simulink model "attitude_kalman_filter"  (R2023a)
settings: configuration reference "configuration_filter" (kept outside this file)
undefined symbols (not defined in the file): alignment_done_bool, dead_reckoning_bool, DiscIntNeverNeededParam, Eul_rad, filt, lin_acc_est_mDs2, rot_K_est_bias_OB_B_radDs, rot_K_est_OB_B_radDs, sfor_est_B_mDs, sfor_est_bias_B_mDs2, sim, x_est
libraries: lib_jacobians x5, lib_kinematics x4
settings Model: Creator=FC_dev1  LastModifiedBy=FC_dev1
settings ConfigSetRef: SourceName=configuration_filter  SourceLocation=Base Workspace

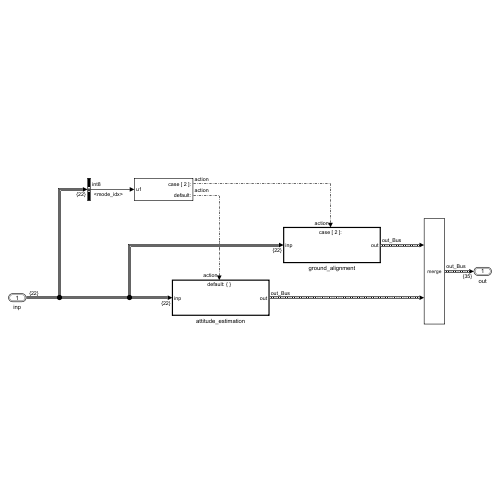
[thumbnail: Simulink's stored preview of the top-level diagram]
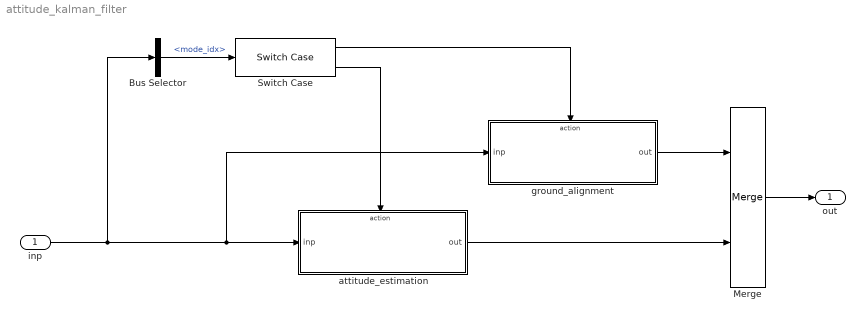
== system attitude_kalman_filter ==
  inp : Inport  OutDataTypeStr=Bus: inp_Bus
  Bus Selector : BusSelector  OutputSignals=mode_idx
  Merge : Merge
  Switch Case : SwitchCase  CaseConditions={filt.modes.ground_alignment}
  attitude_estimation : Subsystem
  ground_alignment : Subsystem
  out : Outport  OutDataTypeStr=Bus: out_Bus
  wires:
  inp/1 -> Bus Selector/1, attitude_estimation/1(inp), ground_alignment/1(inp)
  attitude_estimation/1(out) -> Merge/2
  Bus Selector/1 -> Switch Case/1  "<mode_idx>"
  Switch Case/1 -> ground_alignment/Action
  Switch Case/2 -> attitude_estimation/Action
  ground_alignment/1(out) -> Merge/1
  Merge/1 -> out/1

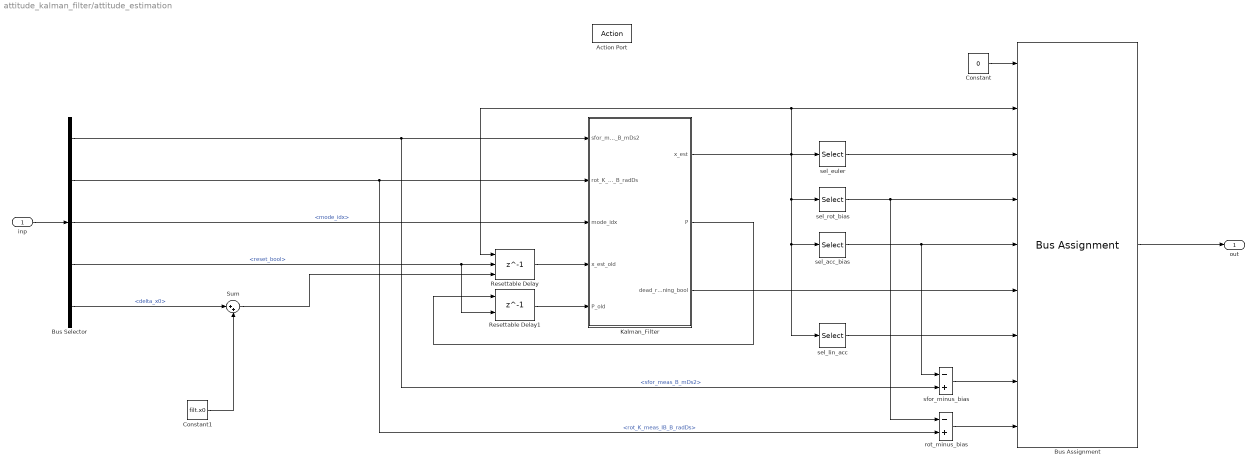
== system attitude_kalman_filter/attitude_estimation ==
  inp : Inport  OutDataTypeStr=Bus: inp_Bus
  Action Port : ActionPort  InitializeStates=reset  ActionPortLabel=default:
  Bus Assignment : BusAssignment  AssignedSignals=x_est,Eul_rad,rot_K_est_bias_OB_B_radDs,sfor_est_bias_B_mDs2,dead_reckoning_bool,lin_acc_est_mDs2,sfor_est_B_mDs,rot_K_est_OB_B_radDs
  Bus Selector : BusSelector  OutputSignals=sfor_meas_B_mDs2,rot_K_meas_IB_B_radDs,mode_idx,reset_bool,delta_x0
  Constant : Constant  Value=0  OutDataTypeStr=Bus: out_Bus
  Constant1 : Constant  Value=filt.x0  VectorParams1D=off
  Kalman_Filter : Subsystem
  Resettable Delay : Delay  DelayLength=1  InitialConditionSource=Input port  ExternalReset=Level hold
      settings: InputPortMap=u0,r5,p4
  Resettable Delay1 : Delay  DelayLength=1  InitialCondition=filt.P0  ExternalReset=Level hold
      settings: InputPortMap=u0,r5
  Sum : Sum  Inputs=|++
  rot_minus_bias : Sum  Inputs=-+
  sel_acc_bias : Selector  NumberOfDimensions=2  InputPortWidth=3  IndexOptions=Index vector (dialog),Index vector (dialog)  Indices=filt.acc_bias_idx,1  OutputSizes=1,1
  sel_euler : Selector  NumberOfDimensions=2  InputPortWidth=3  IndexOptions=Index vector (dialog),Index vector (dialog)  Indices=filt.eul_idx,1  OutputSizes=1,1
  sel_lin_acc : Selector  NumberOfDimensions=2  InputPortWidth=3  IndexOptions=Index vector (dialog),Index vector (dialog)  Indices=filt.lin_acc_idx,1  OutputSizes=1,1
  sel_rot_bias : Selector  NumberOfDimensions=2  InputPortWidth=3  IndexOptions=Index vector (dialog),Index vector (dialog)  Indices=filt.rot_bias_idx,1  OutputSizes=1,1
  sfor_minus_bias : Sum  Inputs=-+
  out : Outport  OutDataTypeStr=Bus: out_Bus
  wires:
  Bus Selector/1 -> sfor_minus_bias/2, Kalman_Filter/1(sfor_meas_B_mDs2)  "<sfor_meas_B_mDs2>"
  rot_minus_bias/1 -> Bus Assignment/9
  sel_acc_bias/1 -> sfor_minus_bias/1, Bus Assignment/5
  sel_rot_bias/1 -> rot_minus_bias/1, Bus Assignment/4
  Bus Selector/2 -> rot_minus_bias/2, Kalman_Filter/2(rot_K_meas_IB_B_radDs)  "<rot_K_meas_IB_B_radDs>"
  Constant/1 -> Bus Assignment/1
  Bus Selector/3 -> Kalman_Filter/3(mode_idx)  "<mode_idx>"
  sel_euler/1 -> Bus Assignment/3
  Kalman_Filter/1(x_est) -> sel_lin_acc/1, sel_acc_bias/1, sel_rot_bias/1, Resettable Delay/1, Bus Assignment/2, sel_euler/1
  Bus Assignment/1 -> out/1
  sel_lin_acc/1 -> Bus Assignment/7
  sfor_minus_bias/1 -> Bus Assignment/8
  Kalman_Filter/3(dead_reckoning_bool) -> Bus Assignment/6
  inp/1 -> Bus Selector/1
  Resettable Delay1/1 -> Kalman_Filter/5(P_old)
  Resettable Delay/1 -> Kalman_Filter/4(x_est_old)
  Bus Selector/4 -> Resettable Delay1/2, Resettable Delay/2  "<reset_bool>"
  Bus Selector/5 -> Sum/1  "<delta_x0>"
  Kalman_Filter/2(P) -> Resettable Delay1/1
  Sum/1 -> Resettable Delay/3
  Constant1/1 -> Sum/2

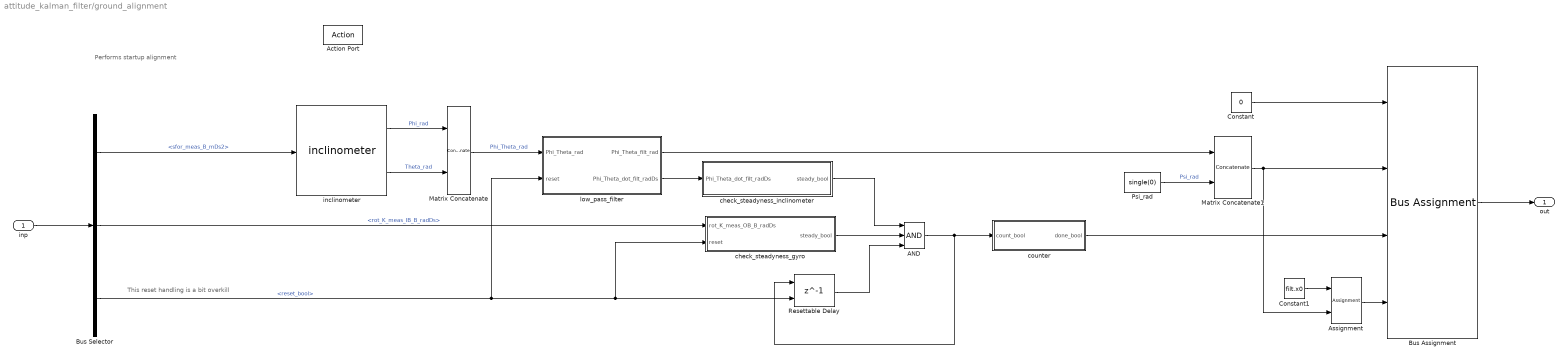
== system attitude_kalman_filter/ground_alignment ==
  note: Performs startup alignment
  note: This reset handling is a bit overkill
  inp : Inport  OutDataTypeStr=Bus: inp_Bus
  Action Port : ActionPort  InitializeStates=reset  ActionPortLabel=case [ 2 ]:
  AND : Logic  Inputs=3  AllPortsSameDT=off  OutDataTypeStr=boolean
  Assignment : Assignment  NumberOfDimensions=2  DiagnosticForDimensions=Warning  IndexOptions=Index vector (dialog),Index vector (dialog)  Indices=filt.eul_idx,1  OutputSizes=1,1
  Bus Assignment : BusAssignment  AssignedSignals=Eul_rad,alignment_done_bool,x_est
  Bus Selector : BusSelector  OutputSignals=sfor_meas_B_mDs2,rot_K_meas_IB_B_radDs,reset_bool
  Constant : Constant  Value=0  OutDataTypeStr=Bus: out_Bus
  Constant1 : Constant  Value=filt.x0  VectorParams1D=off
  Matrix Concatenate : Concatenate  Mode=Multidimensional array
  Matrix Concatenate1 : Concatenate  Mode=Multidimensional array
  Psi_rad : Constant  Value=single(0)
  Resettable Delay : Delay  DelayLength=1  InitialCondition=false  ExternalReset=Level
      settings: InputPortMap=u0,r5
  check_steadyness_gyro : Subsystem
  check_steadyness_inclinometer : Subsystem
  counter : Subsystem
  inclinometer : lib_kinematics/inclinometer  SystemSampleTime=-1  VariantActivationTime=update diagram  Latency=0  AutoFrameSizeCalculation=off
  low_pass_filter : Subsystem
  out : Outport  OutDataTypeStr=Bus: out_Bus
  wires:
  inp/1 -> Bus Selector/1
  Bus Assignment/1 -> out/1
  Constant/1 -> Bus Assignment/1
  Bus Selector/1 -> inclinometer/1  "<sfor_meas_B_mDs2>"
  inclinometer/2 -> Matrix Concatenate/2  "Theta_rad"
  inclinometer/1 -> Matrix Concatenate/1  "Phi_rad"
  Psi_rad/1 -> Matrix Concatenate1/2  "Psi_rad"
  Matrix Concatenate/1 -> low_pass_filter/1(Phi_Theta_rad)  "Phi_Theta_rad"
  low_pass_filter/1(Phi_Theta_filt_rad) -> Matrix Concatenate1/1
  Matrix Concatenate1/1 -> Bus Assignment/2, Assignment/2
  low_pass_filter/2(Phi_Theta_dot_filt_radDs) -> check_steadyness_inclinometer/1(Phi_Theta_dot_filt_radDs)
  Bus Selector/2 -> check_steadyness_gyro/1(rot_K_meas_OB_B_radDs)  "<rot_K_meas_IB_B_radDs>"
  check_steadyness_inclinometer/1(steady_bool) -> AND/1
  check_steadyness_gyro/1(steady_bool) -> AND/2
  AND/1 -> counter/1(count_bool), Resettable Delay/1
  counter/1(done_bool) -> Bus Assignment/3
  Bus Selector/3 -> low_pass_filter/2(reset), check_steadyness_gyro/2(reset), Resettable Delay/2  "<reset_bool>"
  Resettable Delay/1 -> AND/3
  Assignment/1 -> Bus Assignment/4
  Constant1/1 -> Assignment/1

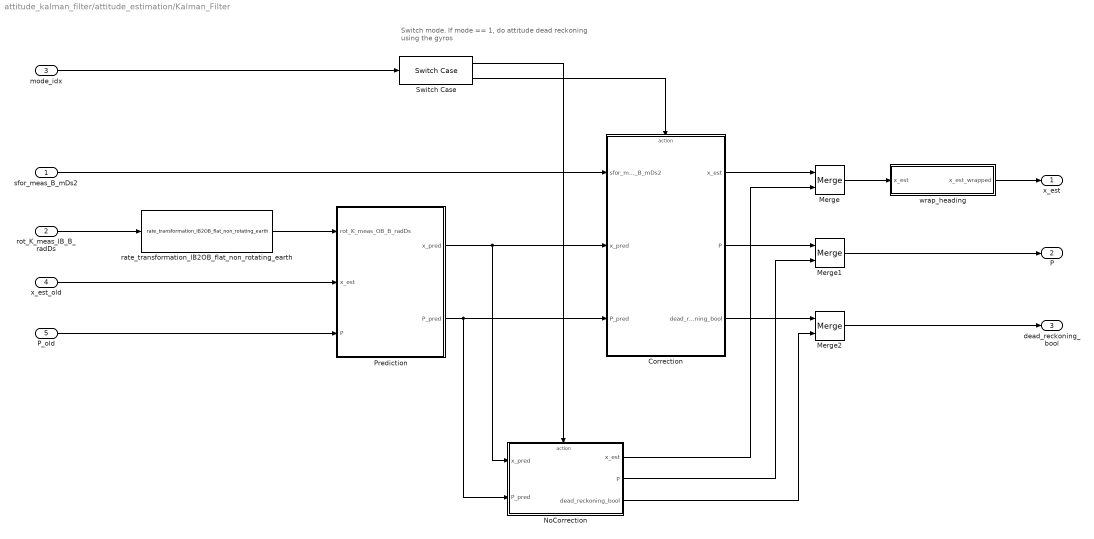
== system attitude_kalman_filter/attitude_estimation/Kalman_Filter ==
  note: Switch mode.
      | If mode == 1, do attitude dead reckoning using the gyros
  sfor_meas_B_mDs2 : Inport
  rot_K_meas_IB_B_radDs : Inport  Port=2
  mode_idx : Inport  Port=3
  x_est_old : Inport  Port=4
  P_old : Inport  Port=5
  Correction : Subsystem
  Merge : Merge
  Merge1 : Merge
  Merge2 : Merge
  NoCorrection : Subsystem
  Prediction : Subsystem
  Switch Case : SwitchCase  CaseConditions={filt.modes.dead_reckoning}
  rate_transformation_IB2OB_flat_non_rotating_earth : lib_kinematics/rate_transformation_IB2OB_flat_non_rotating_earth  SystemSampleTime=-1  VariantActivationTime=update diagram  Latency=0  AutoFrameSizeCalculation=off
  wrap_heading : Subsystem
  x_est : Outport
  P : Outport  Port=2
  dead_reckoning_bool : Outport  Port=3
  wires:
  Prediction/2(P_pred) -> Correction/3(P_pred), NoCorrection/2(P_pred)
  x_est_old/1 -> Prediction/2(x_est)
  Correction/2(P) -> Merge1/1
  sfor_meas_B_mDs2/1 -> Correction/1(sfor_meas_B_mDs2)
  Prediction/1(x_pred) -> NoCorrection/1(x_pred), Correction/2(x_pred)
  rot_K_meas_IB_B_radDs/1 -> rate_transformation_IB2OB_flat_non_rotating_earth/1
  Correction/1(x_est) -> Merge/1
  P_old/1 -> Prediction/3(P)
  mode_idx/1 -> Switch Case/1
  Switch Case/1 -> NoCorrection/Action
  Merge/1 -> wrap_heading/1(x_est)
  Merge1/1 -> P/1
  Switch Case/2 -> Correction/Action
  NoCorrection/1(x_est) -> Merge/2
  NoCorrection/2(P) -> Merge1/2
  Merge2/1 -> dead_reckoning_bool/1
  Correction/3(dead_reckoning_bool) -> Merge2/1
  NoCorrection/3(dead_reckoning_bool) -> Merge2/2
  rate_transformation_IB2OB_flat_non_rotating_earth/1 -> Prediction/1(rot_K_meas_OB_B_radDs)
  wrap_heading/1(x_est_wrapped) -> x_est/1

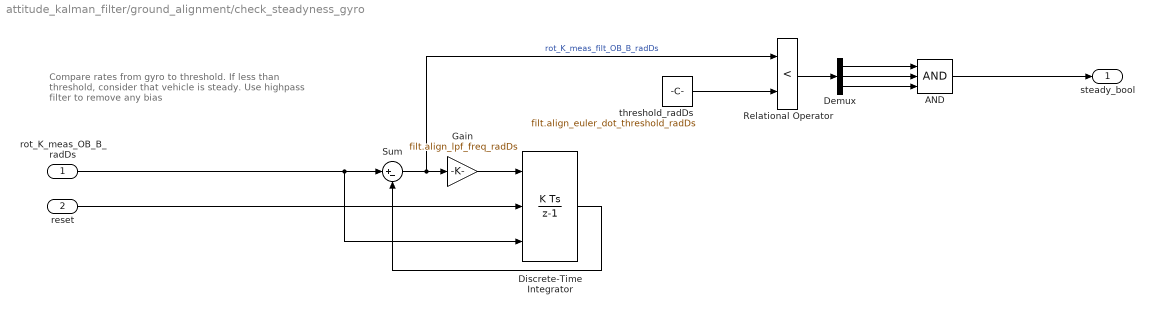
== system attitude_kalman_filter/ground_alignment/check_steadyness_gyro ==
  note: Compare rates from gyro to threshold.
      | If less than threshold, consider that vehicle is steady.
      | Use highpass filter to remove any bias
  rot_K_meas_OB_B_radDs : Inport
  reset : Inport  Port=2
  AND : Logic  Inputs=3  AllPortsSameDT=off  OutDataTypeStr=boolean
  Demux : Demux  Outputs=3
  Discrete-Time Integrator : DiscreteIntegrator  ExternalReset=level  InitialConditionSource=external  SampleTime=sim.sample_time_s  ICPrevOutput=DiscIntNeverNeededParam  ICPrevScaledInput=DiscIntNeverNeededParam
  Gain : Gain  Gain=filt.align_lpf_freq_radDs
  Relational Operator : RelationalOperator  Operator=<  OutDataTypeStr=boolean  RndMeth=Simplest  InputSameDT=off
  Sum : Sum  Inputs=|+-
  threshold_radDs : Constant  Value=filt.align_euler_dot_threshold_radDs
  steady_bool : Outport
  wires:
  threshold_radDs/1 -> Relational Operator/2
  Gain/1 -> Discrete-Time Integrator/1
  Discrete-Time Integrator/1 -> Sum/2
  rot_K_meas_OB_B_radDs/1 -> Sum/1, Discrete-Time Integrator/3
  Sum/1 -> Relational Operator/1, Gain/1  "rot_K_meas_filt_OB_B_radDs"
  Demux/2 -> AND/2
  Demux/1 -> AND/1
  Relational Operator/1 -> Demux/1
  AND/1 -> steady_bool/1
  Demux/3 -> AND/3
  reset/1 -> Discrete-Time Integrator/2

== system attitude_kalman_filter/ground_alignment/check_steadyness_inclinometer ==
  note: Compare euler_dot from inclinometer to threshold.
      | If less than threshold, consider that vehicle is steady.
  Phi_Theta_dot_filt_radDs : Inport
  AND : Logic  AllPortsSameDT=off  OutDataTypeStr=boolean
  Demux : Demux  Outputs=2
  Relational Operator : RelationalOperator  Operator=<  OutDataTypeStr=boolean  RndMeth=Simplest  InputSameDT=off
  threshold_radDs : Constant  Value=filt.align_euler_dot_threshold_radDs
  steady_bool : Outport
  wires:
  Phi_Theta_dot_filt_radDs/1 -> Relational Operator/1
  threshold_radDs/1 -> Relational Operator/2
  Relational Operator/1 -> Demux/1
  Demux/1 -> AND/1
  Demux/2 -> AND/2
  AND/1 -> steady_bool/1

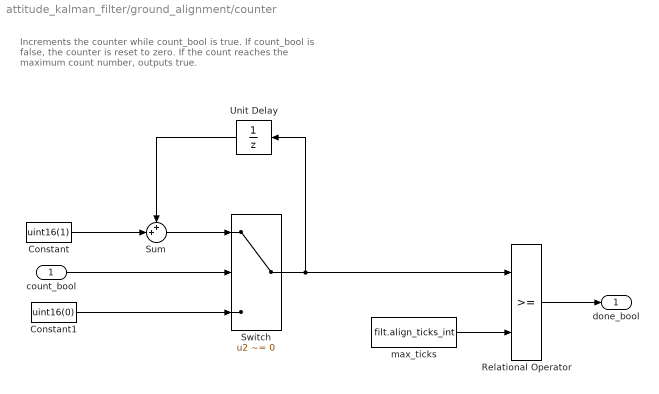
== system attitude_kalman_filter/ground_alignment/counter ==
  note: Increments the counter while count_bool is true.
      | If count_bool is false, the counter is reset to zero.
      | If the count reaches the maximum count number, outputs true.
  count_bool : Inport
  Constant : Constant  Value=uint16(1)
  Constant1 : Constant  Value=uint16(0)
  Relational Operator : RelationalOperator  OutDataTypeStr=boolean  RndMeth=Simplest  InputSameDT=off
  Sum : Sum  Inputs=++|
  Switch : Switch  Criteria=u2 ~= 0  SaturateOnIntegerOverflow=off  InputSameDT=off
  Unit Delay : UnitDelay  InitialCondition=uint16(0)  SampleTime=-1  HasFrameUpgradeWarning=on
  max_ticks : Constant  Value=filt.align_ticks_int
  done_bool : Outport
  wires:
  Relational Operator/1 -> done_bool/1
  max_ticks/1 -> Relational Operator/2
  count_bool/1 -> Switch/2
  Constant/1 -> Sum/2
  Constant1/1 -> Switch/3
  Switch/1 -> Relational Operator/1, Unit Delay/1
  Unit Delay/1 -> Sum/1
  Sum/1 -> Switch/1

== system attitude_kalman_filter/ground_alignment/low_pass_filter ==
  Phi_Theta_rad : Inport
  reset : Inport  Port=2
  Discrete-Time Integrator : DiscreteIntegrator  ExternalReset=level  InitialConditionSource=external  SampleTime=sim.sample_time_s  ICPrevOutput=DiscIntNeverNeededParam  ICPrevScaledInput=DiscIntNeverNeededParam
  Gain : Gain  Gain=filt.align_lpf_freq_radDs
  Sum : Sum  Inputs=|+-
  Phi_Theta_filt_rad : Outport
  Phi_Theta_dot_filt_radDs : Outport  Port=2
  wires:
  Phi_Theta_rad/1 -> Discrete-Time Integrator/3, Sum/1
  Sum/1 -> Gain/1
  Discrete-Time Integrator/1 -> Phi_Theta_filt_rad/1, Sum/2
  Gain/1 -> Phi_Theta_dot_filt_radDs/1, Discrete-Time Integrator/1
  reset/1 -> Discrete-Time Integrator/2

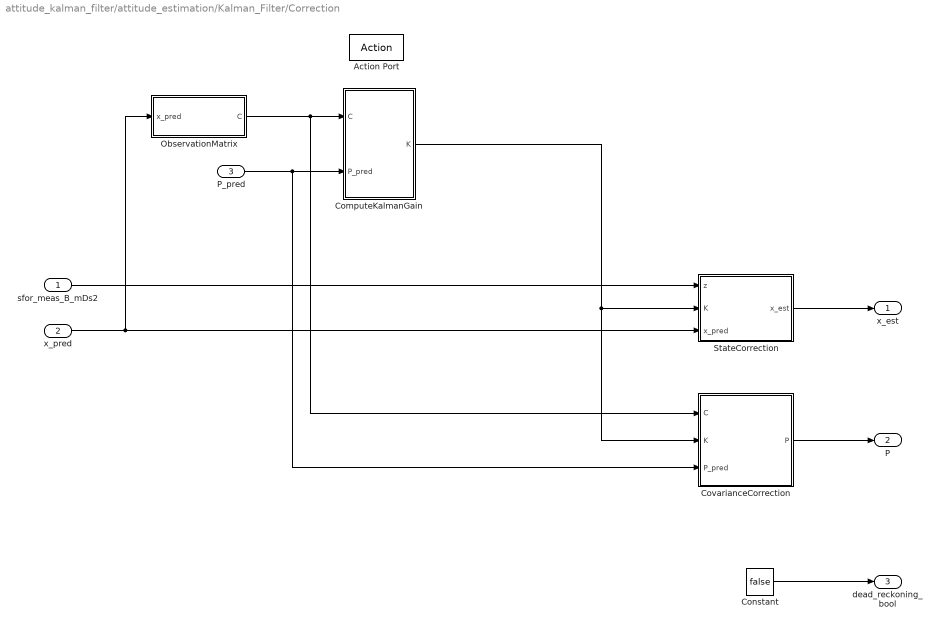
== system attitude_kalman_filter/attitude_estimation/Kalman_Filter/Correction ==
  sfor_meas_B_mDs2 : Inport
  x_pred : Inport  Port=2
  P_pred : Inport  Port=3
  Action Port : ActionPort  ActionPortLabel=default:
  ComputeKalmanGain : Subsystem
  Constant : Constant  Value=false
  CovarianceCorrection : Subsystem
  ObservationMatrix : Subsystem
  StateCorrection : Subsystem
  x_est : Outport
  P : Outport  Port=2
  dead_reckoning_bool : Outport  Port=3
  wires:
  P_pred/1 -> CovarianceCorrection/3(P_pred), ComputeKalmanGain/2(P_pred)
  ObservationMatrix/1(C) -> CovarianceCorrection/1(C), ComputeKalmanGain/1(C)
  StateCorrection/1(x_est) -> x_est/1
  CovarianceCorrection/1(P) -> P/1
  x_pred/1 -> ObservationMatrix/1(x_pred), StateCorrection/3(x_pred)
  ComputeKalmanGain/1(K) -> CovarianceCorrection/2(K), StateCorrection/2(K)
  sfor_meas_B_mDs2/1 -> StateCorrection/1(z)
  Constant/1 -> dead_reckoning_bool/1

== system attitude_kalman_filter/attitude_estimation/Kalman_Filter/NoCorrection ==
  note: Bypass correction step.
      | Just to test dead reckoning.
  x_pred : Inport
  P_pred : Inport  Port=2
  Action Port : ActionPort  ActionPortLabel=case [ 1 ]:
  Constant : Constant  Value=true
  x_est : Outport
  P : Outport  Port=2
  dead_reckoning_bool : Outport  Port=3
  wires:
  P_pred/1 -> P/1
  x_pred/1 -> x_est/1
  Constant/1 -> dead_reckoning_bool/1

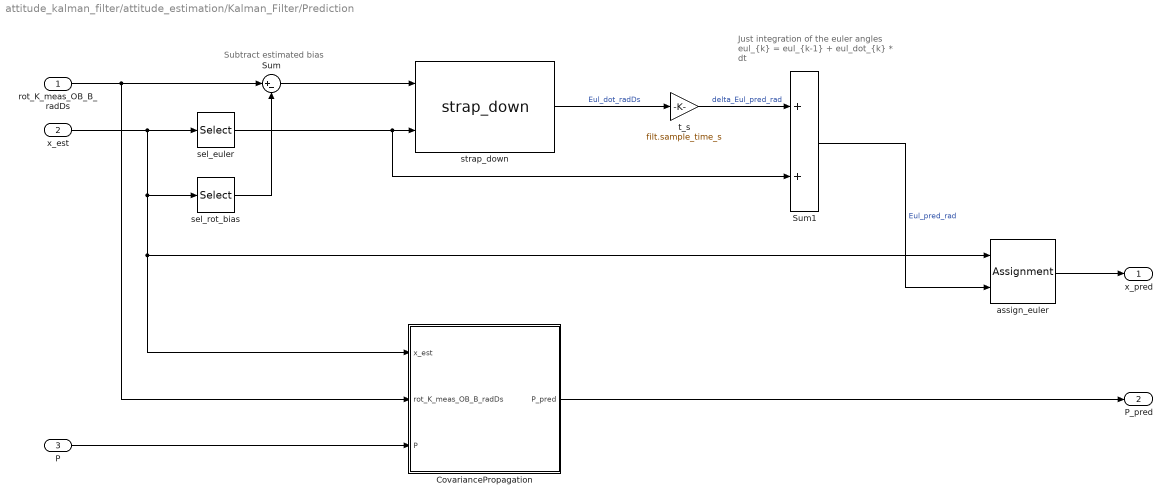
== system attitude_kalman_filter/attitude_estimation/Kalman_Filter/Prediction ==
  note: Just integration of the euler angles
      | eul_{k} = eul_{k-1} + eul_dot_{k} * dt
  note: Subtract estimated bias
  rot_K_meas_OB_B_radDs : Inport
  x_est : Inport  Port=2
  P : Inport  Port=3
  CovariancePropagation : Subsystem
  Sum : Sum  Inputs=|+-
  Sum1 : Sum
  assign_euler : Assignment  NumberOfDimensions=2  DiagnosticForDimensions=Warning  IndexOptions=Index vector (dialog),Index vector (dialog)  Indices=filt.eul_idx,1  OutputSizes=1,1
  sel_euler : Selector  NumberOfDimensions=2  InputPortWidth=3  IndexOptions=Index vector (dialog),Index vector (dialog)  Indices=filt.eul_idx,1  OutputSizes=1,1
  sel_rot_bias : Selector  NumberOfDimensions=2  InputPortWidth=3  IndexOptions=Index vector (dialog),Index vector (dialog)  Indices=filt.rot_bias_idx,1  OutputSizes=1,1
  strap_down : lib_kinematics/strap_down  SystemSampleTime=-1  VariantActivationTime=update diagram  Latency=0  AutoFrameSizeCalculation=off
  t_s : Gain  Gain=filt.sample_time_s
  x_pred : Outport
  P_pred : Outport  Port=2
  wires:
  rot_K_meas_OB_B_radDs/1 -> CovariancePropagation/2(rot_K_meas_OB_B_radDs), Sum/1
  x_est/1 -> CovariancePropagation/1(x_est), assign_euler/1, sel_rot_bias/1, sel_euler/1
  P/1 -> CovariancePropagation/3(P)
  CovariancePropagation/1(P_pred) -> P_pred/1
  sel_euler/1 -> Sum1/2, strap_down/2
  Sum/1 -> strap_down/1
  sel_rot_bias/1 -> Sum/2
  strap_down/1 -> t_s/1  "Eul_dot_radDs"
  t_s/1 -> Sum1/1  "delta_Eul_pred_rad"
  Sum1/1 -> assign_euler/2  "Eul_pred_rad"
  assign_euler/1 -> x_pred/1

== system attitude_kalman_filter/attitude_estimation/Kalman_Filter/wrap_heading ==
  x_est : Inport
  Assignment : Assignment  NumberOfDimensions=2  DiagnosticForDimensions=Warning  IndexOptions=Index vector (dialog),Index vector (dialog)  Indices=filt.eul_idx(3),1  OutputSizes=1,1
  Terminator : Terminator
  sel_psi : Selector  NumberOfDimensions=2  InputPortWidth=3  IndexOptions=Index vector (dialog),Index vector (dialog)  Indices=filt.eul_idx(3),1  OutputSizes=1,1
  wrap_0_360 : lib_kinematics/wrap_0_360  SystemSampleTime=-1  VariantActivationTime=update diagram  Latency=0  AutoFrameSizeCalculation=off
  x_est_wrapped : Outport
  wires:
  x_est/1 -> sel_psi/1, Assignment/1
  sel_psi/1 -> wrap_0_360/1  "psi_est_rad"
  Assignment/1 -> x_est_wrapped/1
  wrap_0_360/1 -> Assignment/2
  wrap_0_360/2 -> Terminator/1

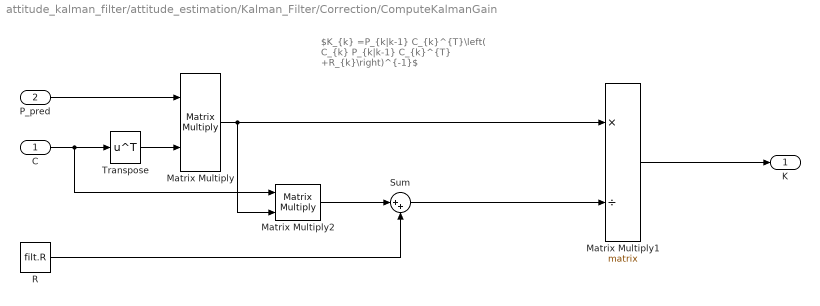
== system attitude_kalman_filter/attitude_estimation/Kalman_Filter/Correction/ComputeKalmanGain ==
  note: $K_{k} =P_{k|k-1} C_{k}^{T}\left( C_{k} P_{k|k-1} C_{k}^{T} +R_{k}\right)^{-1}$
  C : Inport
  P_pred : Inport  Port=2
  Matrix Multiply : Product  Multiplication=Matrix(*)
  Matrix Multiply1 : Product  Inputs=*/  Multiplication=Matrix(*)
  Matrix Multiply2 : Product  Multiplication=Matrix(*)
  R : Constant  Value=filt.R  VectorParams1D=off
  Sum : Sum  Inputs=|++
  Transpose : Math  Operator=transpose
  K : Outport
  wires:
  P_pred/1 -> Matrix Multiply/1
  C/1 -> Matrix Multiply2/1, Transpose/1
  Transpose/1 -> Matrix Multiply/2
  Matrix Multiply2/1 -> Sum/1
  Sum/1 -> Matrix Multiply1/2
  R/1 -> Sum/2
  Matrix Multiply1/1 -> K/1
  Matrix Multiply/1 -> Matrix Multiply2/2, Matrix Multiply1/1

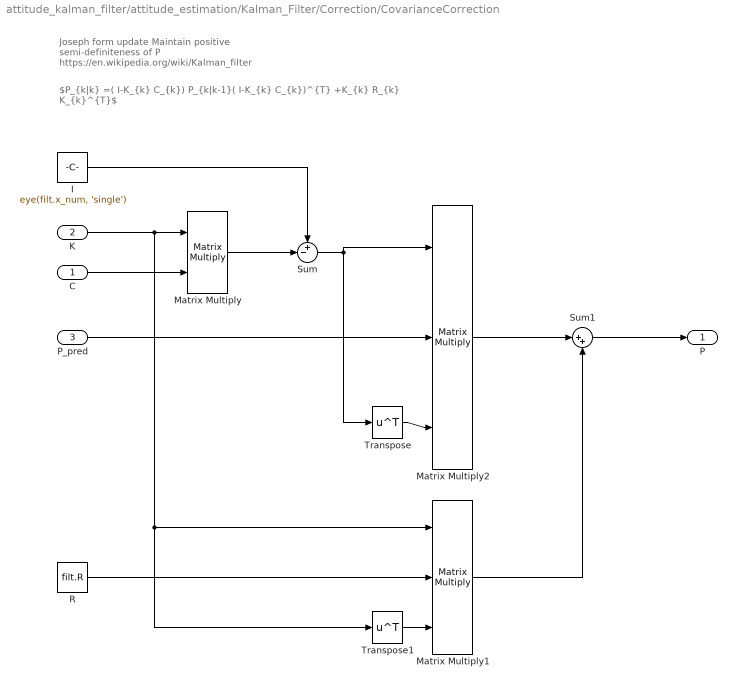
== system attitude_kalman_filter/attitude_estimation/Kalman_Filter/Correction/CovarianceCorrection ==
  note: $P_{k|k} =( I-K_{k} C_{k}) P_{k|k-1}( I-K_{k} C_{k})^{T} +K_{k} R_{k} K_{k}^{T}$
  note: Joseph form update
      | Maintain positive semi-definiteness of P
      | https://en.wikipedia.org/wiki/Kalman_filter
  C : Inport
  K : Inport  Port=2
  P_pred : Inport  Port=3
  I : Constant  Value=eye(filt.x_num, 'single')  VectorParams1D=off
  Matrix Multiply : Product  Multiplication=Matrix(*)
  Matrix Multiply1 : Product  Inputs=3  Multiplication=Matrix(*)
  Matrix Multiply2 : Product  Inputs=3  Multiplication=Matrix(*)
  R : Constant  Value=filt.R  VectorParams1D=off
  Sum : Sum  Inputs=+-|
  Sum1 : Sum  Inputs=|++
  Transpose : Math  Operator=transpose
  Transpose1 : Math  Operator=transpose
  P : Outport
  wires:
  C/1 -> Matrix Multiply/2
  K/1 -> Transpose1/1, Matrix Multiply1/1, Matrix Multiply/1
  Matrix Multiply/1 -> Sum/2
  Sum1/1 -> P/1
  I/1 -> Sum/1
  Sum/1 -> Transpose/1, Matrix Multiply2/1
  P_pred/1 -> Matrix Multiply2/2
  Transpose/1 -> Matrix Multiply2/3
  Transpose1/1 -> Matrix Multiply1/3
  R/1 -> Matrix Multiply1/2
  Matrix Multiply1/1 -> Sum1/2
  Matrix Multiply2/1 -> Sum1/1

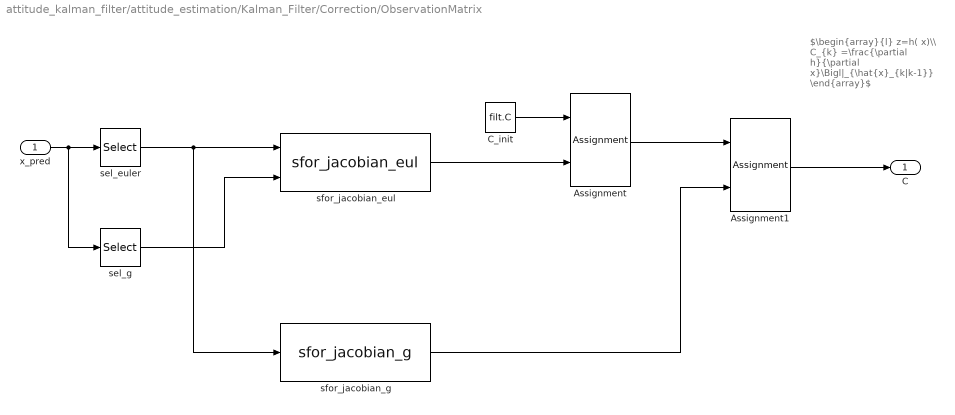
== system attitude_kalman_filter/attitude_estimation/Kalman_Filter/Correction/ObservationMatrix ==
  note: $\begin{array}{l} z=h( x)\\ C_{k} =\frac{\partial h}{\partial x}\Bigl|_{\hat{x}_{k|k-1}} \end{array}$
  x_pred : Inport
  Assignment : Assignment  NumberOfDimensions=2  DiagnosticForDimensions=Warning  IndexOptions=Assign all,Index vector (dialog)  Indices=1,filt.eul_idx  OutputSizes=1,1
  Assignment1 : Assignment  NumberOfDimensions=2  DiagnosticForDimensions=Warning  IndexOptions=Assign all,Index vector (dialog)  Indices=1,filt.g_idx  OutputSizes=1,1
  C_init : Constant  Value=filt.C  VectorParams1D=off
  sel_euler : Selector  NumberOfDimensions=2  InputPortWidth=3  IndexOptions=Index vector (dialog),Index vector (dialog)  Indices=filt.eul_idx,1  OutputSizes=1,1
  sel_g : Selector  NumberOfDimensions=2  InputPortWidth=3  IndexOptions=Index vector (dialog),Index vector (dialog)  Indices=filt.g_idx,1  OutputSizes=1,1
  sfor_jacobian_eul : lib_jacobians/sfor_jacobian_eul  SystemSampleTime=-1  VariantActivationTime=update diagram  Latency=0  AutoFrameSizeCalculation=off
  sfor_jacobian_g : lib_jacobians/sfor_jacobian_g  SystemSampleTime=-1  VariantActivationTime=update diagram  Latency=0  AutoFrameSizeCalculation=off
  C : Outport
  wires:
  x_pred/1 -> sel_g/1, sel_euler/1
  sel_euler/1 -> sfor_jacobian_eul/1, sfor_jacobian_g/1
  sel_g/1 -> sfor_jacobian_eul/2
  C_init/1 -> Assignment/1
  sfor_jacobian_eul/1 -> Assignment/2
  Assignment/1 -> Assignment1/1
  Assignment1/1 -> C/1
  sfor_jacobian_g/1 -> Assignment1/2

== system attitude_kalman_filter/attitude_estimation/Kalman_Filter/Correction/StateCorrection ==
  note: $\hat{x}_{k|k} =\hat{x}_{k|k-1} +K_{k}( z_{k} -h(\hat{x}_{k|k-1}))$
  z : Inport
  K : Inport  Port=2
  x_pred : Inport  Port=3
  Matrix Multiply : Product  Multiplication=Matrix(*)
  Sum : Sum  Inputs=|++
  Sum1 : Sum  Inputs=|+-
  observation_function : Subsystem
  x_est : Outport
  wires:
  x_pred/1 -> observation_function/1(x_pred), Sum/1
  K/1 -> Matrix Multiply/1
  Matrix Multiply/1 -> Sum/2
  Sum/1 -> x_est/1
  z/1 -> Sum1/1
  observation_function/1(h_x_pred) -> Sum1/2
  Sum1/1 -> Matrix Multiply/2

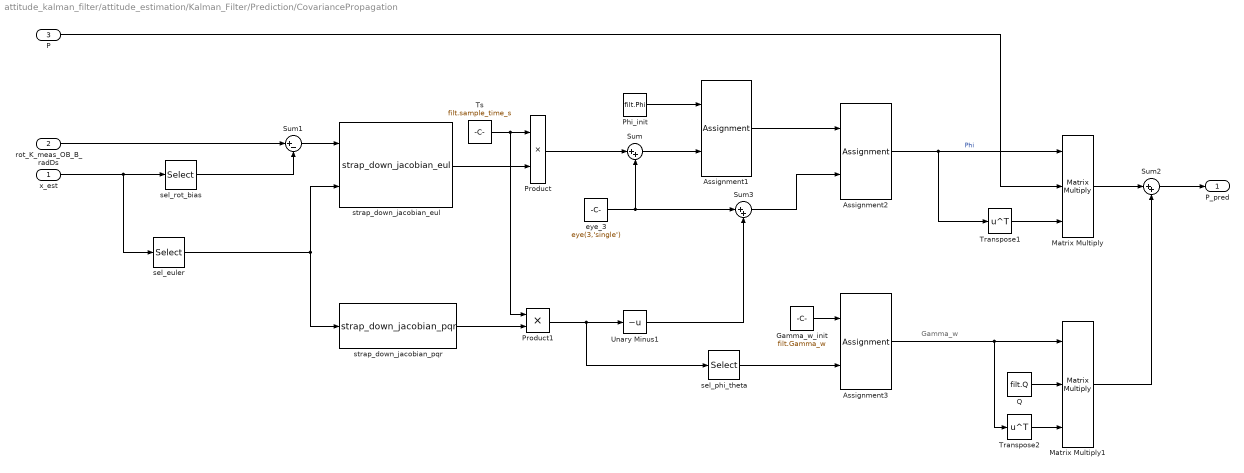
== system attitude_kalman_filter/attitude_estimation/Kalman_Filter/Prediction/CovariancePropagation ==
  note: Gamma_w
  x_est : Inport
  rot_K_meas_OB_B_radDs : Inport  Port=2
  P : Inport  Port=3
  Assignment1 : Assignment  NumberOfDimensions=2  DiagnosticForDimensions=Warning  IndexOptions=Index vector (dialog),Index vector (dialog)  Indices=filt.eul_idx,filt.eul_idx  OutputSizes=1,1
  Assignment2 : Assignment  NumberOfDimensions=2  DiagnosticForDimensions=Warning  IndexOptions=Index vector (dialog),Index vector (dialog)  Indices=filt.rot_bias_idx,filt.rot_bias_idx  OutputSizes=1,1
  Assignment3 : Assignment  NumberOfDimensions=2  DiagnosticForDimensions=Warning  IndexOptions=Index vector (dialog),Index vector (dialog)  Indices=filt.eul_idx(1:2),filt.rot_noise_idx  OutputSizes=1,1
  Gamma_w_init : Constant  Value=filt.Gamma_w  VectorParams1D=off
  Matrix Multiply : Product  Inputs=3  Multiplication=Matrix(*)
  Matrix Multiply1 : Product  Inputs=3  Multiplication=Matrix(*)
  Phi_init : Constant  Value=filt.Phi  VectorParams1D=off
  Product : Product
  Product1 : Product
  Q : Constant  Value=filt.Q  VectorParams1D=off
  Sum : Sum  Inputs=|++
  Sum1 : Sum  Inputs=|+-
  Sum2 : Sum  Inputs=|++
  Sum3 : Sum  Inputs=|++
  Transpose1 : Math  Operator=transpose
  Transpose2 : Math  Operator=transpose
  Ts : Constant  Value=filt.sample_time_s
  Unary Minus1 : UnaryMinus
  eye_3 : Constant  Value=eye(3,'single')  VectorParams1D=off
  sel_euler : Selector  NumberOfDimensions=2  InputPortWidth=3  IndexOptions=Index vector (dialog),Index vector (dialog)  Indices=filt.eul_idx,1  OutputSizes=1,1
  sel_phi_theta : Selector  NumberOfDimensions=2  InputPortWidth=3  IndexOptions=Index vector (dialog),Select all  Indices=[1 2],1  OutputSizes=1,1
  sel_rot_bias : Selector  NumberOfDimensions=2  InputPortWidth=3  IndexOptions=Index vector (dialog),Index vector (dialog)  Indices=filt.rot_bias_idx,1  OutputSizes=1,1
  strap_down_jacobian_eul : lib_jacobians/strap_down_jacobian_eul  SystemSampleTime=-1  VariantActivationTime=update diagram  Latency=0  AutoFrameSizeCalculation=off
  strap_down_jacobian_pqr : lib_jacobians/strap_down_jacobian_pqr  SystemSampleTime=-1  VariantActivationTime=update diagram  Latency=0  AutoFrameSizeCalculation=off
  P_pred : Outport
  wires:
  P/1 -> Matrix Multiply/2
  Transpose1/1 -> Matrix Multiply/3
  x_est/1 -> sel_rot_bias/1, sel_euler/1
  sel_euler/1 -> strap_down_jacobian_eul/2, strap_down_jacobian_pqr/1
  rot_K_meas_OB_B_radDs/1 -> Sum1/1
  sel_rot_bias/1 -> Sum1/2
  strap_down_jacobian_eul/1 -> Product/2
  Product/1 -> Sum/1
  Phi_init/1 -> Assignment1/1
  Sum/1 -> Assignment1/2
  eye_3/1 -> Sum3/1, Sum/2
  strap_down_jacobian_pqr/1 -> Product1/2
  Sum1/1 -> strap_down_jacobian_eul/1
  Product1/1 -> Unary Minus1/1, sel_phi_theta/1
  Assignment1/1 -> Assignment2/1
  Unary Minus1/1 -> Sum3/2
  Gamma_w_init/1 -> Assignment3/1
  Assignment2/1 -> Matrix Multiply/1, Transpose1/1  "Phi"
  Assignment3/1 -> Transpose2/1, Matrix Multiply1/1
  Transpose2/1 -> Matrix Multiply1/3
  Q/1 -> Matrix Multiply1/2
  Matrix Multiply/1 -> Sum2/1
  Sum2/1 -> P_pred/1
  Matrix Multiply1/1 -> Sum2/2
  Ts/1 -> Product1/1, Product/1
  Sum3/1 -> Assignment2/2
  sel_phi_theta/1 -> Assignment3/2

== system attitude_kalman_filter/attitude_estimation/Kalman_Filter/Correction/StateCorrection/observation_function ==
  x_pred : Inport
  Product : Product
  Sum : Sum  Inputs=+++
  sel_acc_bias : Selector  NumberOfDimensions=2  InputPortWidth=3  IndexOptions=Index vector (dialog),Index vector (dialog)  Indices=filt.acc_bias_idx,1  OutputSizes=1,1
  sel_eul : Selector  NumberOfDimensions=2  InputPortWidth=3  IndexOptions=Index vector (dialog),Index vector (dialog)  Indices=filt.eul_idx,1  OutputSizes=1,1
  sel_g : Selector  NumberOfDimensions=2  InputPortWidth=3  IndexOptions=Index vector (dialog),Index vector (dialog)  Indices=filt.g_idx,1  OutputSizes=1,1
  sel_lin_acc : Selector  NumberOfDimensions=2  InputPortWidth=3  IndexOptions=Index vector (dialog),Index vector (dialog)  Indices=filt.lin_acc_idx,1  OutputSizes=1,1
  sfor_jacobian_g : lib_jacobians/sfor_jacobian_g  SystemSampleTime=-1  VariantActivationTime=update diagram  Latency=0  AutoFrameSizeCalculation=off
  h_x_pred : Outport
  wires:
  x_pred/1 -> sel_lin_acc/1, sel_acc_bias/1, sel_g/1, sel_eul/1
  Sum/1 -> h_x_pred/1
  sel_acc_bias/1 -> Sum/2  "acc_bias"
  sel_eul/1 -> sfor_jacobian_g/1
  sfor_jacobian_g/1 -> Product/1
  sel_g/1 -> Product/2
  Product/1 -> Sum/1  "acc_g"
  sel_lin_acc/1 -> Sum/3  "lin_acc"
